simulink model "Target_Control_System"  (R2021b)
settings: Solver=FixedStepDiscrete  StartTime=0.0  StopTime=5  RelTol=1e-3
PreLoadFcn:
  | RTWConfigurationCB('preloadfcn', bdroot);
PostLoadFcn:
  | load('configuration/data_struct.mat');
  | load('configuration/fluxMaps_propMotor.mat');
  | load('configuration/parameterInit_PROP.mat');
  | load('configuration/parameterInit_PUMP.mat');
  | load('configuration/parameterInit_PITCH.mat');
  | load('configuration/parameterInit_TILT.mat');
  | %load('configuration/base_workspace_signal_definition.mat');
  | %load('resolvedatastores_to_baseworkspace_for_faster_simulation.mat');
model workspace (MAT data in the model file):
  SIMULATION_OPTIONS : Simulink.Parameter (value not decoded)
  TARGET_CODE_GEN : Simulink.Parameter (value not decoded)
  TCS_SAMPLE_FREQ_HZ : Simulink.Parameter (value not decoded)
symbols that are objects in the model workspace (value not decoded): TARGET_CODE_GEN, TCS_SAMPLE_FREQ_HZ
undefined symbols (not defined in the file): A_DQ_REF_LPF_INIT__PITCH, A_DQ_REF_LPF_INIT__PROP, A_DQ_REF_LPF_INIT__PUMP, A_DQ_REF_LPF_INIT__TILT, A_OBSERVER_CONFIDENCE_INIT__PITCH, A_OBSERVER_CONFIDENCE_INIT__PROP, A_OBSERVER_CONFIDENCE_INIT__PUMP, A_OBSERVER_CONFIDENCE_INIT__TILT, ACTUATOR_MAX_ANGLE_TRIP__PITCH, ACTUATOR_MIN_ANGLE_TRIP__PITCH, ACTUATOR_POS_SENSOR_INV_DIRECTION__PITCH, ACTUATOR_POS_SENSOR_INV_DIRECTION__TILT, ACTUATOR_POS_SENSOR_OFFSET__PITCH, ACTUATOR_POS_SENSOR_OFFSET__TILT, ADC_scaler1_baseaddr_TILT, ADC_SCALER_FLOAT_TO_FIXPOINT_EXPANSION, ANGLE_ELEC_FROM_SENSOR_OFFSET_INIT__PITCH, ANGLE_ELEC_FROM_SENSOR_OFFSET_INIT__PROP, ANGLE_ELEC_FROM_SENSOR_OFFSET_INIT__PUMP, ANGLE_ELEC_FROM_SENSOR_OFFSET_INIT__TILT, AUTO_CLEAR_FAULTS_ENABLED__PITCH, AUTO_CLEAR_FAULTS_ENABLED__PROP, AUTO_CLEAR_FAULTS_ENABLED__PUMP, AUTO_CLEAR_FAULTS_ENABLED__TILT, AUTO_CLEAR_FAULTS_WAIT_TICKS__PITCH, AUTO_CLEAR_FAULTS_WAIT_TICKS__PROP, AUTO_CLEAR_FAULTS_WAIT_TICKS__PUMP, AUTO_CLEAR_FAULTS_WAIT_TICKS__TILT, AUTO_I_ZERO_IDLE_TICKS__PITCH, AUTO_I_ZERO_IDLE_TICKS__PROP, AUTO_I_ZERO_IDLE_TICKS__PUMP, AUTO_I_ZERO_IDLE_TICKS__TILT, AUTO_I_ZERO_OFFSET_IDC_THRESHOLD__PITCH, AUTO_I_ZERO_OFFSET_IDC_THRESHOLD__PROP, AUTO_I_ZERO_OFFSET_IDC_THRESHOLD__PUMP, AUTO_I_ZERO_OFFSET_IDC_THRESHOLD__TILT, AUTO_I_ZERO_OFFSET_IPH_THRESHOLD__PITCH, AUTO_I_ZERO_OFFSET_IPH_THRESHOLD__PROP, AUTO_I_ZERO_OFFSET_IPH_THRESHOLD__PUMP, AUTO_I_ZERO_OFFSET_IPH_THRESHOLD__TILT, AUTO_SENSORLESS_SWITCHOVER_DISABLE_OMEGA, AUTO_SENSORLESS_SWITCHOVER_ENABLE_OMEGA, AUTO_SENSORLESS_SWITCHOVER_MIN_CONFIDENCE, AUXILIARY_PROTECTION_UNIT_BASEADDR__TILT, blanking_max_error_omega_INIT_PITCH, blanking_max_error_omega_INIT_TILT, blanking_max_error_position_INIT_PITCH, blanking_max_error_position_INIT_TILT, BRUTE_START_I_Q_REF_RAMP_SPEED__PITCH, BRUTE_START_I_Q_REF_RAMP_SPEED__PROP, BRUTE_START_I_Q_REF_RAMP_SPEED__PUMP, BRUTE_START_I_Q_REF_RAMP_SPEED__TILT, CONTROL_LOOP_DT_INIT__PITCH, CONTROL_LOOP_DT_INIT__PROP, CONTROL_LOOP_DT_INIT__PUMP, CONTROL_LOOP_DT_INIT__TILT, CORRECTION_FILTER_SCALE__PITCH, CORRECTION_FILTER_SCALE__PROP, CORRECTION_FILTER_SCALE__PUMP, CORRECTION_FILTER_SCALE__TILT ... (+458)
libraries: simulink x178, Reusables_Lib x24
(part 19 of 47)

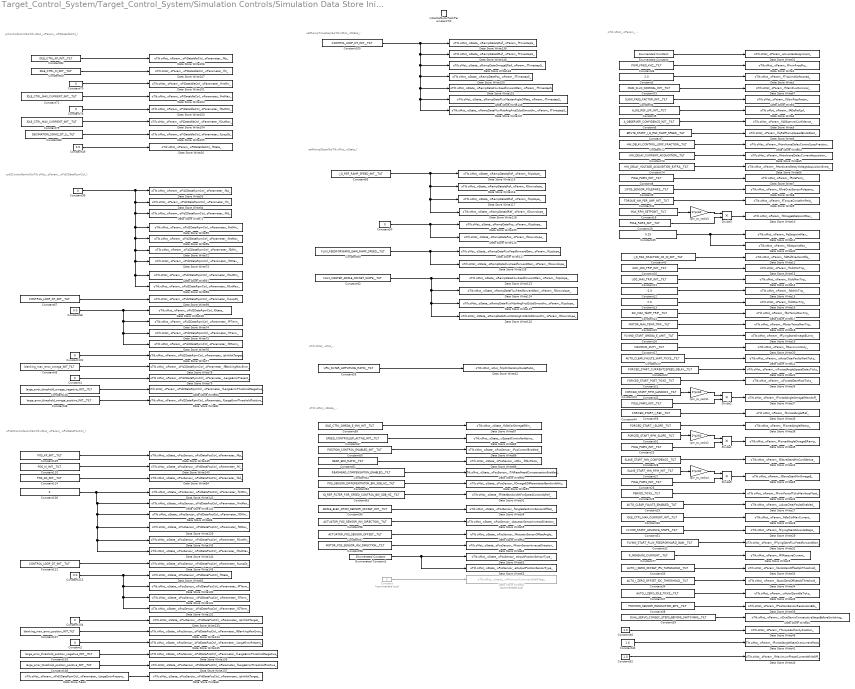
== system Target_Control_System/Target_Control_System/Simulation Controls/Simulation Data Store Initialization/initializeDataForTilt()/initializeMotorTaskParametersTilt ==
  note: oTilt.oMot_.oState_...
  note: oTilt.oMot_.oParam_...
  note: oTilt.oMot_.oOut_...
  note: setRampSlope(&oTilt.oMot_.oState_)
  note: setRampTimestep(&oTilt.oMot_.oState_)
  note: oPid2ControllerInit(&oTilt.oMot_.oParam_.oPidDataPosCtrl_)
  note: pid2ControllerInit(&oTilt.oMot_.oParam_.oPid2DataRpmCtrl_)
  note: piControllerInit(&oTilt.oMot_.oParam_.oPiDataIdleCtrl_)
  initializeMotorTaskParametersTilt : TriggerPort  TriggerType=function-call  VariantControl=Variant
  Constant : Constant  Commented=on  Value=0  OutDataTypeStr=uint32  SampleTime=-1
  Constant{1..2,101,104} (4 alike) : Constant  Value=0  OutDataTypeStr=int32  SampleTime=-1
  Constant10 : Constant  Value=UDC_MIN_TRIP_INIT__TILT  OutDataTypeStr=single  SampleTime=-1
  Constant100 : Constant  Value=large_error_threshold_omega_negative_INIT__ITLT  OutDataTypeStr=single  SampleTime=-1
  Constant103 : Constant  Value=large_error_threshold_position_negative_INIT__ITLT  OutDataTypeStr=single  SampleTime=-1
  Constant105 : Constant  Value=CONTROL_LOOP_DT_INIT__TILT  OutDataTypeStr=single  SampleTime=-1
  Constant{50,70,78,99,106} (5 alike) : Constant  Value=0  OutDataTypeStr=single  SampleTime=-1
  Constant107 : Constant  Value=blanking_max_error_position_INIT_TILT  OutDataTypeStr=single  SampleTime=-1
  Constant108 : Constant  Value=large_error_threshold_position_positive_INIT__TILT  OutDataTypeStr=single  SampleTime=-1
  Constant109 : Constant  Value=POS_KP_INIT__TILT  OutDataTypeStr=single  SampleTime=-1
  Constant11 : Constant  Value=UDC_MAX_TRIP_INIT__TILT  VectorParams1D=off  OutDataTypeStr=single  SampleTime=-1
  Constant110 : Constant  Value=POS_KI_INIT__TILT  OutDataTypeStr=single  SampleTime=-1
  Constant112 : Constant  Value=CONTROL_LOOP_DT_INIT__TILT  OutDataTypeStr=single  SampleTime=-1
  Constant113 : Constant  Value=0.0  OutDataTypeStr=single  SampleTime=-1
  Constant114 : Constant  Value=POS_KD_INIT__TILT  OutDataTypeStr=single  SampleTime=-1
  Constant12 : Constant  Value=-2.0  OutDataTypeStr=single  SampleTime=-1
  Constant13 : Constant  Value=2.0  OutDataTypeStr=single  SampleTime=-1
  Constant14 : Constant  Value=SIC_MAX_TEMP_TRIP__TILT  OutDataTypeStr=single  SampleTime=-1
  Constant15 : Constant  Value=MOTOR_MAX_TEMP_TRIP__TILT  OutDataTypeStr=single  SampleTime=-1
  Constant16 : Constant  Value=FLYING_START_OMEGA_E_LIMIT__TILT  OutDataTypeStr=single  SampleTime=-1
  Constant17 : Constant  Value=MAXIMUM_DUTY__TILT  VectorParams1D=off  OutDataTypeStr=single  SampleTime=-1
  Constant18 : Constant  Value=MAX_RPM_SETPOINT__TILT  OutDataTypeStr=single  SampleTime=-1
  Constant{8,19,23..24,26} (5 alike) : Constant  Value=POLE_PAIRS_INIT__TILT  OutDataTypeStr=single  SampleTime=-1
  Constant20 : Constant  Value=AUTO_CLEAR_FAULTS_WAIT_TICKS__TILT  OutDataTypeStr=uint32  SampleTime=-1
  Constant21 : Constant  Value=FORCED_START_POST_TICKS__TILT  OutDataTypeStr=uint32  SampleTime=-1
  Constant22 : Constant  Value=FORCED_START_CURRENT2SPEED_DELAY__TILT  OutDataTypeStr=uint32  SampleTime=-1
  Constant25 : Constant  Value=PERIOD_TICKS__TILT  OutDataTypeStr=single  SampleTime=-1
  Constant27 : Constant  Value=SLAVE_START_MIN_RPM_INIT__TILT  OutDataTypeStr=single  SampleTime=-1
  Constant28 : Constant  Value=SLAVE_START_MIN_CONFIDENCE__TILT  OutDataTypeStr=single  SampleTime=-1
  Constant29 : Constant  Value=AUTO_CLEAR_FAULTS_ENABLED__TILT  OutDataTypeStr=uint32  SampleTime=-1
  Constant3 : Constant  Value=2.0  OutDataTypeStr=single  SampleTime=-1
  Constant30 : Constant  Value=IDLE_CTRL_MAX_CURRENT_INIT__TILT  OutDataTypeStr=single  SampleTime=-1
  Constant31 : Constant  Value=FLYING_START_ADVANCE_STEPS__TILT  OutDataTypeStr=single  SampleTime=-1
  Constant32 : Constant  Value=FLYING_START_FLUX_FEEDFORWARD_GAIN__TILT  OutDataTypeStr=single  SampleTime=-1
  Constant33 : Constant  Value=AUTO_I_ZERO_OFFSET_IPH_THRESHOLD__TILT  OutDataTypeStr=single  SampleTime=-1
  Constant34 : Constant  Value=AUTO_I_ZERO_OFFSET_IDC_THRESHOLD__TILT  VectorParams1D=off  OutDataTypeStr=single  SampleTime=-1
  Constant35 : Constant  Value=0.25  VectorParams1D=off  OutDataTypeStr=single  SampleTime=-1
  Constant36 : Constant  Value=PWM_FREQ_KHZ__TILT  OutDataTypeStr=single  SampleTime=-1
  Constant37 : Constant  Value=AUTO_I_ZERO_IDLE_TICKS__TILT  OutDataTypeStr=uint32  SampleTime=-1
  Constant38 : Constant  Value=POSITION_SENSOR_RESOLUTION_BITS__TILT  OutDataTypeStr=single  SampleTime=-1
  Constant39 : Constant  Value=DUAL_SERVO_CONSEC_STEPS_BEFORE_SWITCHING__TILT  OutDataTypeStr=uint32  SampleTime=-1
  Constant4 : Constant  Value=SLOW_PASS_FACTOR_INIT__TILT  OutDataTypeStr=single  SampleTime=-1
  Constant40 : Constant  Value=1.6  OutDataTypeStr=single  SampleTime=-1
  Constant41 : Constant  Value=TORQUE_NM_PER_AMP_INIT__TILT  VectorParams1D=off  OutDataTypeStr=single  SampleTime=-1
  Constant42 : Constant  Value=FORCED_START_RPM_HANDOFF__TILT  OutDataTypeStr=single  SampleTime=-1
  Constant43 : Constant  Value=I_D_REF_FRACTION_OF_IQ_INIT__TILT  OutDataTypeStr=single  SampleTime=-1
  Constant44 : Constant  Value=FORCED_START_I_SLOPE__TILT  OutDataTypeStr=single  SampleTime=-1
  Constant45 : Constant  Value=blanking_max_error_omega_INIT_TILT  OutDataTypeStr=single  SampleTime=-1
  Constant46 : Constant  Value=1.0  OutDataTypeStr=single  SampleTime=-1
  Constant47 : Constant  Value=SPEED_CONTROLLER_ACTIVE_INIT__TILT  OutDataTypeStr=uint32  SampleTime=-1
  Constant48 : Constant  Value=large_error_threshold_omega_positive_INIT__TILT  OutDataTypeStr=single  SampleTime=-1
  Constant49 : Constant  Value=0.0  OutDataTypeStr=single  SampleTime=-1
  Constant5 : Constant  Value=A_DQ_REF_LPF_INIT__TILT  OutDataTypeStr=single  SampleTime=-1
  Constant51 : Constant  Value=FORCED_START_RPM_SLOPE__TILT  OutDataTypeStr=single  SampleTime=-1
  Constant52 : Constant  Value=1.0  OutDataTypeStr=single  SampleTime=-1
  Constant55 : Constant  Value=UPH_FILTER_AMPLITUDE_RATIO__TILT  VectorParams1D=off  OutDataTypeStr=single  SampleTime=-1
  Constant56 : Constant  Value=FORCED_START_I_REF__TILT  VectorParams1D=off  OutDataTypeStr=single  SampleTime=-1
  Constant58 : Constant  Value=IDLE_CTRL_OMEGA_E_MIN_INIT__TILT  OutDataTypeStr=single  SampleTime=-1
  Constant6 : Constant  Value=A_OBSERVER_CONFIDENCE_INIT__TILT  OutDataTypeStr=single  SampleTime=-1
  Constant60 : Constant  Value=POSITION_CONTROL_ENABLED_INIT__TILT  OutDataTypeStr=int32  SampleTime=-1
  Constant61 : Constant  Value=GEAR_BOX_RATIO__TILT  OutDataTypeStr=single  SampleTime=-1
  Constant62 : Constant  Value=READHEAD_COMPENSATION_ENABLED__TILT  OutDataTypeStr=int32  SampleTime=-1
  Constant63 : Constant  Value=IQ_REF_FILTER_FOR_SPEED_CONTROL_BW_3DB_HZ__TILT  OutDataTypeStr=single  SampleTime=-1
  Constant67 : Constant  Value=CONTROL_LOOP_DT_INIT__TILT  OutDataTypeStr=single  SampleTime=-1
  Constant68 : Constant  Value=0.0  OutDataTypeStr=single  SampleTime=-1
  Constant69 : Constant  Value=IDLE_CTRL_KI_INIT__TILT  OutDataTypeStr=single  SampleTime=-1
  Constant7 : Constant  Value=BRUTE_START_I_Q_REF_RAMP_SPEED__TILT  OutDataTypeStr=single  SampleTime=-1
  Constant71 : Constant  Value=IDLE_CTRL_MAX_CURRENT_INIT__TILT  OutDataTypeStr=single  SampleTime=-1
  Constant72 : Constant  Value=HW_DELAY_CONTROL_LOOP_FRACTION__TILT  OutDataTypeStr=single  SampleTime=-1
  Constant73 : Constant  Value=HW_DELAY_CURRENT_ACQUISITION__TILT  OutDataTypeStr=single  SampleTime=-1
  Constant74 : Constant  Value=HW_DELAY_VOLTAGE_ACQUISITION_EXTRA__TILT  OutDataTypeStr=single  SampleTime=-1
  Constant75 : Constant  Value=MAIN_FLUX_NOMINAL_INIT__TILT  OutDataTypeStr=single  SampleTime=-1
  Constant77 : Constant  Value=R_MEASURE_CURRENT__TILT  OutDataTypeStr=single  SampleTime=-1
  Constant79 : Constant  Value=IDLE_CTRL_MAX_CURRENT_INIT__TILT  VectorParams1D=off  OutDataTypeStr=single  SampleTime=-1
  Constant80 : Constant  Value=DECIMATION_200HZ_DT_S__TILT  OutDataTypeStr=single  SampleTime=-1
  Constant81 : Constant  Value=IDLE_CTRL_KP_INIT__TILT  OutDataTypeStr=single  SampleTime=-1
  Constant83 : Constant  Value=I_Q_REF_RAMP_SPEED_INIT__TILT  OutDataTypeStr=single  SampleTime=-1
  Constant89 : Constant  Value=FLUX_FEEDFORWARD_GAIN_RAMP_SPEED__TILT  OutDataTypeStr=single  SampleTime=-1
  Constant9 : Constant  Value=1/POS_SENSOR_POLEPAIRS__TILT  OutDataTypeStr=single  SampleTime=-1
  Constant92 : Constant  Value=FLUX_MASTER_ANGLE_OFFSET_SLOPE__TILT  OutDataTypeStr=single  SampleTime=-1
  Constant94 : Constant  Value=POS_SENSOR_DIFFERENTIATOR_BW_3DB_HZ__TILT  OutDataTypeStr=single  SampleTime=-1
  Constant95 : Constant  Value=ANGLE_ELEC_FROM_SENSOR_OFFSET_INIT__TILT  OutDataTypeStr=single  SampleTime=-1
  Constant96 : Constant  Value=ACTUATOR_POS_SENSOR_INV_DIRECTION__TILT  OutDataTypeStr=int32  SampleTime=-1
  Constant97 : Constant  Value=ACTUATOR_POS_SENSOR_OFFSET__TILT  OutDataTypeStr=single  SampleTime=-1
  Constant98 : Constant  Value=MOTOR_POS_SENSOR_INV_DIRECTION__TILT  OutDataTypeStr=int32  SampleTime=-1
  Data Store Read : DataStoreRead  DataStoreName=oTilt  DataStoreElements=oTilt.oMot_.oParam_.oPid2DataRpmCtrl_.oParameter_.iLargeErrorPresent_  IndexOptions=Index vector (dialog)  Indices=1  OutputSizes=1
  Data Store Write1 : DataStoreWrite  DataStoreName=oTilt  DataStoreElements=oTilt.oMot_.oParam_.fPwmFreqKhz_  IndexOptions=Index vector (dialog)  Indices=1  OutputSizes=1
  Data Store Write10 : DataStoreWrite  DataStoreName=oTilt  DataStoreElements=oTilt.oMot_.oParam_.fOmegaESetpointMax_  IndexOptions=Index vector (dialog)  Indices=1  OutputSizes=1
  Data Store Write100 : DataStoreWrite  DataStoreName=oTilt  DataStoreElements=oTilt.oMot_.oParam_.oPid2DataRpmCtrl_.fState_  IndexOptions=Index vector (dialog)  Indices=1  OutputSizes=1
  Data Store Write101 : DataStoreWrite  DataStoreName=oTilt  DataStoreElements=oTilt.oMot_.oParam_.oPiDataIdleCtrl_.oParameter_.fIntMin_  IndexOptions=Index vector (dialog)  Indices=1  OutputSizes=1
  Data Store Write102 : DataStoreWrite  DataStoreName=oTilt  DataStoreElements=oTilt.oMot_.oParam_.oPiDataIdleCtrl_.oParameter_.fIntMax_  IndexOptions=Index vector (dialog)  Indices=1  OutputSizes=1
  Data Store Write103 : DataStoreWrite  DataStoreName=oTilt  DataStoreElements=oTilt.oMot_.oParam_.oPiDataIdleCtrl_.oParameter_.fOutMin_  IndexOptions=Index vector (dialog)  Indices=1  OutputSizes=1
  Data Store Write104 : DataStoreWrite  DataStoreName=oTilt  DataStoreElements=oTilt.oMot_.oParam_.oPiDataIdleCtrl_.oParameter_.fOutMax_  IndexOptions=Index vector (dialog)  Indices=1  OutputSizes=1
  Data Store Write105 : DataStoreWrite  DataStoreName=oTilt  DataStoreElements=oTilt.oMot_.oParam_.oPiDataIdleCtrl_.oParameter_.fLoopDt_  IndexOptions=Index vector (dialog)  Indices=1  OutputSizes=1
  Data Store Write106 : DataStoreWrite  DataStoreName=oTilt  DataStoreElements=oTilt.oMot_.oParam_.oPiDataIdleCtrl_.oParameter_.fKp_  IndexOptions=Index vector (dialog)  Indices=1  OutputSizes=1
  Data Store Write107 : DataStoreWrite  DataStoreName=oTilt  DataStoreElements=oTilt.oMot_.oParam_.oPiDataIdleCtrl_.oParameter_.fKi_  IndexOptions=Index vector (dialog)  Indices=1  OutputSizes=1
  Data Store Write11 : DataStoreWrite  DataStoreName=oTilt  DataStoreElements=oTilt.oMot_.oParam_.fIqSetpointMax_  IndexOptions=Index vector (dialog)  Indices=1  OutputSizes=1
  Data Store Write115 : DataStoreWrite  DataStoreName=oTilt  DataStoreElements=oTilt.oMot_.oState_.oRampDataIqRef_.oParam_.fUpslope_  IndexOptions=Index vector (dialog)  Indices=1  OutputSizes=1
  Data Store Write116 : DataStoreWrite  DataStoreName=oTilt  DataStoreElements=oTilt.oMot_.oState_.oRampDataIqRef_.oParam_.fDownslope_  IndexOptions=Index vector (dialog)  Indices=1  OutputSizes=1
  Data Store Write117 : DataStoreWrite  DataStoreName=oTilt  DataStoreElements=oTilt.oMot_.oState_.oRampDataIdRef_.oParam_.fUpslope_  IndexOptions=Index vector (dialog)  Indices=1  OutputSizes=1
  Data Store Write118 : DataStoreWrite  DataStoreName=oTilt  DataStoreElements=oTilt.oMot_.oState_.oRampDataIdRef_.oParam_.fDownslope_  IndexOptions=Index vector (dialog)  Indices=1  OutputSizes=1
  Data Store Write119 : DataStoreWrite  DataStoreName=oTilt  DataStoreElements=oTilt.oMot_.oState_.oRampDataFluxMstrAngFrcd2clsdSmoothn_.oParam_.fUpslope_  IndexOptions=Index vector (dialog)  Indices=1  OutputSizes=1
  Data Store Write12 : DataStoreWrite  DataStoreName=oTilt  DataStoreElements=oTilt.oMot_.oParam_.fIdRefFractionOfIq_  IndexOptions=Index vector (dialog)  Indices=1  OutputSizes=1
  Data Store Write120 : DataStoreWrite  DataStoreName=oTilt  DataStoreElements=oTilt.oMot_.oState_.oRampDataFluxMstrAngFrcd2clsdSmoothn_.oParam_.fDownslope_  IndexOptions=Index vector (dialog)  Indices=1  OutputSizes=1
  Data Store Write123 : DataStoreWrite  DataStoreName=oTilt  DataStoreElements=oTilt.oMot_.oState_.oRampDataFluxFeedforwardGain_.oParam_.fUpslope_  IndexOptions=Index vector (dialog)  Indices=1  OutputSizes=1
  Data Store Write124 : DataStoreWrite  DataStoreName=oTilt  DataStoreElements=oTilt.oMot_.oState_.oRampDataFluxFeedforwardGain_.oParam_.fDownslope_  IndexOptions=Index vector (dialog)  Indices=1  OutputSizes=1
  Data Store Write125 : DataStoreWrite  DataStoreName=oTilt  DataStoreElements=oTilt.oMot_.oState_.oRampDataPos_.oParam_.fUpslope_  IndexOptions=Index vector (dialog)  Indices=1  OutputSizes=1
  Data Store Write126 : DataStoreWrite  DataStoreName=oTilt  DataStoreElements=oTilt.oMot_.oState_.oRampDataPos_.oParam_.fDownslope_  IndexOptions=Index vector (dialog)  Indices=1  OutputSizes=1
  Data Store Write127 : DataStoreWrite  DataStoreName=oTilt  DataStoreElements=oTilt.oMot_.oState_.oRampDataFluxFeedforwardGain_.oParam_.fUpslope_  IndexOptions=Index vector (dialog)  Indices=1  OutputSizes=1
  Data Store Write128 : DataStoreWrite  DataStoreName=oTilt  DataStoreElements=oTilt.oMot_.oState_.oRampDataFluxFeedforwardGain_.oParam_.fDownslope_  IndexOptions=Index vector (dialog)  Indices=1  OutputSizes=1
  Data Store Write129 : DataStoreWrite  DataStoreName=oTilt  DataStoreElements=oTilt.oMot_.oState_.oPosSensor_.oPidDataPosCtrl_.oParameter_.fDMax_  IndexOptions=Index vector (dialog)  Indices=1  OutputSizes=1
  Data Store Write13 : DataStoreWrite  DataStoreName=oTilt  DataStoreElements=oTilt.oMot_.oParam_.fUdcMinTrip_  IndexOptions=Index vector (dialog)  Indices=1  OutputSizes=1
  Data Store Write130 : DataStoreWrite  DataStoreName=oTilt  DataStoreElements=oTilt.oMot_.oState_.oPosSensor_.oPidDataPosCtrl_.oParameter_.fPTerm_  IndexOptions=Index vector (dialog)  Indices=1  OutputSizes=1
  Data Store Write131 : DataStoreWrite  DataStoreName=oTilt  DataStoreElements=oTilt.oMot_.oState_.oPosSensor_.oPidDataPosCtrl_.oParameter_.fITerm_  IndexOptions=Index vector (dialog)  Indices=1  OutputSizes=1
  Data Store Write132 : DataStoreWrite  DataStoreName=oTilt  DataStoreElements=oTilt.oMot_.oState_.oPosSensor_.oPidDataPosCtrl_.oParameter_.fDTerm_  IndexOptions=Index vector (dialog)  Indices=1  OutputSizes=1
  Data Store Write133 : DataStoreWrite  DataStoreName=oTilt  DataStoreElements=oTilt.oMot_.oState_.oPosSensor_.oPidDataPosCtrl_.oParameter_.ipInhibitTarget_  IndexOptions=Index vector (dialog)  Indices=1  OutputSizes=1
  Data Store Write134 : DataStoreWrite  DataStoreName=oTilt  DataStoreElements=oTilt.oMot_.oState_.oPosSensor_.oPidDataPosCtrl_.oParameter_.fBlankingMaxError_  IndexOptions=Index vector (dialog)  Indices=1  OutputSizes=1
  Data Store Write135 : DataStoreWrite  DataStoreName=oTilt  DataStoreElements=oTilt.oMot_.oState_.oPosSensor_.oPidDataPosCtrl_.oParameter_.iLargeErrorPresent_  IndexOptions=Index vector (dialog)  Indices=1  OutputSizes=1
  Data Store Write136 : DataStoreWrite  DataStoreName=oTilt  DataStoreElements=oTilt.oMot_.oState_.oPosSensor_.oPidDataPosCtrl_.oParameter_.fLargeErrorThresholdNegative_  IndexOptions=Index vector (dialog)  Indices=1  OutputSizes=1
  Data Store Write137 : DataStoreWrite  DataStoreName=oTilt  DataStoreElements=oTilt.oMot_.oState_.oPosSensor_.oPidDataPosCtrl_.oParameter_.fLargeErrorThresholdPositive_  IndexOptions=Index vector (dialog)  Indices=1  OutputSizes=1
  Data Store Write138 : DataStoreWrite  DataStoreName=oTilt  DataStoreElements=oTilt.oMot_.oState_.oRampDataIqRef_.oParam_.fTimestepS_  IndexOptions=Index vector (dialog)  Indices=1  OutputSizes=1
  Data Store Write139 : DataStoreWrite  DataStoreName=oTilt  DataStoreElements=oTilt.oMot_.oState_.oPosSensor_.oPidDataPosCtrl_.oParameter_.fKp_  IndexOptions=Index vector (dialog)  Indices=1  OutputSizes=1
  Data Store Write14 : DataStoreWrite  DataStoreName=oTilt  DataStoreElements=oTilt.oMot_.oParam_.fUdcMaxTrip_  IndexOptions=Index vector (dialog)  Indices=1  OutputSizes=1
  Data Store Write140 : DataStoreWrite  DataStoreName=oTilt  DataStoreElements=oTilt.oMot_.oState_.oPosSensor_.oPidDataPosCtrl_.oParameter_.fKi_  IndexOptions=Index vector (dialog)  Indices=1  OutputSizes=1
  Data Store Write141 : DataStoreWrite  DataStoreName=oTilt  DataStoreElements=oTilt.oMot_.oState_.oPosSensor_.oPidDataPosCtrl_.oParameter_.fIntMin_  IndexOptions=Index vector (dialog)  Indices=1  OutputSizes=1
  Data Store Write142 : DataStoreWrite  DataStoreName=oTilt  DataStoreElements=oTilt.oMot_.oState_.oPosSensor_.oPidDataPosCtrl_.oParameter_.fIntMax_  IndexOptions=Index vector (dialog)  Indices=1  OutputSizes=1
  Data Store Write143 : DataStoreWrite  DataStoreName=oTilt  DataStoreElements=oTilt.oMot_.oState_.oPosSensor_.oPidDataPosCtrl_.oParameter_.fOutMin_  IndexOptions=Index vector (dialog)  Indices=1  OutputSizes=1
  Data Store Write144 : DataStoreWrite  DataStoreName=oTilt  DataStoreElements=oTilt.oMot_.oState_.oPosSensor_.oPidDataPosCtrl_.oParameter_.fOutMax_  IndexOptions=Index vector (dialog)  Indices=1  OutputSizes=1
  Data Store Write145 : DataStoreWrite  DataStoreName=oTilt  DataStoreElements=oTilt.oMot_.oState_.oPosSensor_.oPidDataPosCtrl_.oParameter_.fLoopDt_  IndexOptions=Index vector (dialog)  Indices=1  OutputSizes=1
  Data Store Write146 : DataStoreWrite  DataStoreName=oTilt  DataStoreElements=oTilt.oMot_.oState_.oRampDataIdRef_.oParam_.fTimestepS_  IndexOptions=Index vector (dialog)  Indices=1  OutputSizes=1
  Data Store Write147 : DataStoreWrite  DataStoreName=oTilt  DataStoreElements=oTilt.oMot_.oState_.oRampDataFluxMstrAngFrcd2clsdSmoothn_.oParam_.fTimestepS_  IndexOptions=Index vector (dialog)  Indices=1  OutputSizes=1
  Data Store Write148 : DataStoreWrite  DataStoreName=oTilt  DataStoreElements=oTilt.oMot_.oState_.oRampDataOmegaERef_.oParam_.fTimestepS_  IndexOptions=Index vector (dialog)  Indices=1  OutputSizes=1
  Data Store Write149 : DataStoreWrite  DataStoreName=oTilt  DataStoreElements=oTilt.oMot_.oState_.oRampDataFluxMasterAngleOffset_.oParam_.fTimestepS_  IndexOptions=Index vector (dialog)  Indices=1  OutputSizes=1
  Data Store Write15 : DataStoreWrite  DataStoreName=oTilt  DataStoreElements=oTilt.oMot_.oParam_.fIdcMinTrip_  IndexOptions=Index vector (dialog)  Indices=1  OutputSizes=1
  Data Store Write150 : DataStoreWrite  DataStoreName=oTilt  DataStoreElements=oTilt.oMot_.oState_.oRampDataPos_.oParam_.fTimestepS_  IndexOptions=Index vector (dialog)  Indices=1  OutputSizes=1
  Data Store Write151 : DataStoreWrite  DataStoreName=oTilt  DataStoreElements=oTilt.oMot_.oState_.oRampDataFluxFeedforwardGain_.oParam_.fTimestepS_  IndexOptions=Index vector (dialog)  Indices=1  OutputSizes=1
  Data Store Write16 : DataStoreWrite  DataStoreName=oTilt  DataStoreElements=oTilt.oMot_.oParam_.fIdcMaxTrip_  IndexOptions=Index vector (dialog)  Indices=1  OutputSizes=1
  Data Store Write17 : DataStoreWrite  DataStoreName=oTilt  DataStoreElements=oTilt.oMot_.oParam_.fSicTempMaxTrip_  IndexOptions=Index vector (dialog)  Indices=1  OutputSizes=1
  Data Store Write18 : DataStoreWrite  DataStoreName=oTilt  DataStoreElements=oTilt.oMot_.oParam_.fMotorTempMaxTrip_  IndexOptions=Index vector (dialog)  Indices=1  OutputSizes=1
  Data Store Write19 : DataStoreWrite  DataStoreName=oTilt  DataStoreElements=oTilt.oMot_.oParam_.fFlyingStartOmegaELimit_  IndexOptions=Index vector (dialog)  Indices=1  OutputSizes=1
  Data Store Write2 : DataStoreWrite  DataStoreName=oTilt  DataStoreElements=oTilt.oMot_.oParam_.fTripLimitSoftwareA_  IndexOptions=Index vector (dialog)  Indices=1  OutputSizes=1
  Data Store Write20 : DataStoreWrite  DataStoreName=oTilt  DataStoreElements=oTilt.oMot_.oParam_.fMaximumDuty_  IndexOptions=Index vector (dialog)  Indices=1  OutputSizes=1
  Data Store Write21 : DataStoreWrite  DataStoreName=oTilt  DataStoreElements=oTilt.oMot_.oParam_.uiAutoClearFaultsWaitTicks_  IndexOptions=Index vector (dialog)  Indices=1  OutputSizes=1
  Data Store Write22 : DataStoreWrite  DataStoreName=oTilt  DataStoreElements=oTilt.oMot_.oParam_.uiForcedAngleSpeedDelayTicks_  IndexOptions=Index vector (dialog)  Indices=1  OutputSizes=1
  Data Store Write23 : DataStoreWrite  DataStoreName=oTilt  DataStoreElements=oTilt.oMot_.oParam_.fSlaveStartMinConfidence_  IndexOptions=Index vector (dialog)  Indices=1  OutputSizes=1
  Data Store Write24 : DataStoreWrite  DataStoreName=oTilt  DataStoreElements=oTilt.oMot_.oParam_.fPwmPeriodTicksMainloopFloat_  IndexOptions=Index vector (dialog)  Indices=1  OutputSizes=1
  Data Store Write25 : DataStoreWrite  DataStoreName=oTilt  DataStoreElements=oTilt.oMot_.oParam_.fRMeasureCurrent_  IndexOptions=Index vector (dialog)  Indices=1  OutputSizes=1
  Data Store Write26 : DataStoreWrite  DataStoreName=oTilt  DataStoreElements=oTilt.oMot_.oParam_.oPiDataIdleCtrl_.fState_  IndexOptions=Index vector (dialog)  Indices=1  OutputSizes=1
  Data Store Write27 : DataStoreWrite  DataStoreName=oTilt  DataStoreElements=oTilt.oMot_.oParam_.uiAutoClearFaultsEnabled_  IndexOptions=Index vector (dialog)  Indices=1  OutputSizes=1
  Data Store Write28 : DataStoreWrite  DataStoreName=oTilt  DataStoreElements=oTilt.oMot_.oParam_.fIdleCtrlMaxCurrent_  IndexOptions=Index vector (dialog)  Indices=1  OutputSizes=1
  Data Store Write29 : DataStoreWrite  DataStoreName=oTilt  DataStoreElements=oTilt.oMot_.oParam_.fFlyingStartAdvanceSteps_  IndexOptions=Index vector (dialog)  Indices=1  OutputSizes=1
  Data Store Write3 : DataStoreWrite  DataStoreName=oTilt  DataStoreElements=oTilt.oMot_.oParam_.fSlowPassFactor_  IndexOptions=Index vector (dialog)  Indices=1  OutputSizes=1
  Data Store Write30 : DataStoreWrite  DataStoreName=oTilt  DataStoreElements=oTilt.oMot_.oParam_.fISetpointMax_  IndexOptions=Index vector (dialog)  Indices=1  OutputSizes=1
  Data Store Write31 : DataStoreWrite  DataStoreName=oTilt  DataStoreElements=oTilt.oMot_.oParam_.eInverterAssignment_  IndexOptions=Index vector (dialog)  Indices=1  OutputSizes=1
  Data Store Write32 : DataStoreWrite  DataStoreName=oTilt  DataStoreElements=oTilt.oMot_.oParam_.fFlyingStartFluxFeedforwardGain_  IndexOptions=Index vector (dialog)  Indices=1  OutputSizes=1
  Data Store Write33 : DataStoreWrite  DataStoreName=oTilt  DataStoreElements=oTilt.oMot_.oParam_.fAutoIZeroOffsetIphThreshold_  IndexOptions=Index vector (dialog)  Indices=1  OutputSizes=1
  Data Store Write34 : DataStoreWrite  DataStoreName=oTilt  DataStoreElements=oTilt.oMot_.oParam_.fAutoIZeroOffsetIdcThreshold_  IndexOptions=Index vector (dialog)  Indices=1  OutputSizes=1
  Data Store Write35 : DataStoreWrite  DataStoreName=oTilt  DataStoreElements=oTilt.oMot_.oParam_.uiAutoIZeroIdleTicks_  IndexOptions=Index vector (dialog)  Indices=1  OutputSizes=1
  Data Store Write36 : DataStoreWrite  DataStoreName=oTilt  DataStoreElements=oTilt.oMot_.oParam_.uiForcedStartPostTicks_  IndexOptions=Index vector (dialog)  Indices=1  OutputSizes=1
  Data Store Write37 : DataStoreWrite  DataStoreName=oTilt  DataStoreElements=oTilt.oMot_.oParam_.fForcedAngleOmegaEHandoff_  IndexOptions=Index vector (dialog)  Indices=1  OutputSizes=1
  Data Store Write38 : DataStoreWrite  DataStoreName=oTilt  DataStoreElements=oTilt.oMot_.oParam_.fForcedAngleIRamp_  IndexOptions=Index vector (dialog)  Indices=1  OutputSizes=1
  Data Store Write39 : DataStoreWrite  DataStoreName=oTilt  DataStoreElements=oTilt.oMot_.oParam_.fPositionSensorResolutionBits_  IndexOptions=Index vector (dialog)  Indices=1  OutputSizes=1
  Data Store Write4 : DataStoreWrite  DataStoreName=oTilt  DataStoreElements=oTilt.oMot_.oParam_.fADqRefLpf_  IndexOptions=Index vector (dialog)  Indices=1  OutputSizes=1
  Data Store Write40 : DataStoreWrite  DataStoreName=oTilt  DataStoreElements=oTilt.oMot_.oParam_.uiDualServoConsecutiveStepsBeforeSwitching_  IndexOptions=Index vector (dialog)  Indices=1  OutputSizes=1
  Data Store Write41 : DataStoreWrite  DataStoreName=oTilt  DataStoreElements=oTilt.oMot_.oParam_.fForcedAngleStartOvercurrentRatio_  IndexOptions=Index vector (dialog)  Indices=1  OutputSizes=1
  Data Store Write42 : DataStoreWrite  DataStoreName=oTilt  DataStoreElements=oTilt.oMot_.oOut_.fUphFilterAmplitudeRatio_  IndexOptions=Index vector (dialog)  Indices=1  OutputSizes=1
  Data Store Write43 : DataStoreWrite  DataStoreName=oTilt  DataStoreElements=oTilt.oMot_.oParam_.fMaximumPhaseCurrentWhileOff_  IndexOptions=Index vector (dialog)  Indices=1  OutputSizes=1
  Data Store Write45 : DataStoreWrite  DataStoreName=oTilt  DataStoreElements=oTilt.oMot_.oParam_.fForcedAngleOmegaERamp_  IndexOptions=Index vector (dialog)  Indices=1  OutputSizes=1
  Data Store Write46 : DataStoreWrite  DataStoreName=oTilt  DataStoreElements=oTilt.oMot_.oParam_.fTorqueAuthorityFraction_  IndexOptions=Index vector (dialog)  Indices=1  OutputSizes=1
  Data Store Write49 : DataStoreWrite  DataStoreName=oTilt  DataStoreElements=oTilt.oMot_.oParam_.fForcedAngleIRef_  IndexOptions=Index vector (dialog)  Indices=1  OutputSizes=1
  Data Store Write5 : DataStoreWrite  DataStoreName=oTilt  DataStoreElements=oTilt.oMot_.oParam_.fAObserverConfidence_  IndexOptions=Index vector (dialog)  Indices=1  OutputSizes=1
  Data Store Write55 : DataStoreWrite  DataStoreName=oTilt  DataStoreElements=oTilt.oMot_.oState_.oPosSensor_.fOmegaEDifferentiatorBandwidthHz_  IndexOptions=Index vector (dialog)  Indices=1  OutputSizes=1
  Data Store Write58 : DataStoreWrite  DataStoreName=oTilt  DataStoreElements=oTilt.oMot_.oState_.oPosSensor_.fAngleElecFromSensorOffset_  IndexOptions=Index vector (dialog)  Indices=1  OutputSizes=1
  Data Store Write59 : DataStoreWrite  DataStoreName=oTilt  DataStoreElements=oTilt.oMot_.oState_.oPosSensor_.iActuatorSensorInverseDirection_  IndexOptions=Index vector (dialog)  Indices=1  OutputSizes=1
  Data Store Write6 : DataStoreWrite  DataStoreName=oTilt  DataStoreElements=oTilt.oMot_.oParam_.fIqRefRampSpeedBruteStart_  IndexOptions=Index vector (dialog)  Indices=1  OutputSizes=1
  Data Store Write60 : DataStoreWrite  DataStoreName=oTilt  DataStoreElements=oTilt.oMot_.oState_.oPosSensor_.fActuatorSensorOffsetAngle_  IndexOptions=Index vector (dialog)  Indices=1  OutputSizes=1
  Data Store Write61 : DataStoreWrite  DataStoreName=oTilt  DataStoreElements=oTilt.oMot_.oState_.oPosSensor_.iMotorSensorInverseDirection_  IndexOptions=Index vector (dialog)  Indices=1  OutputSizes=1
  Data Store Write62 : DataStoreWrite  DataStoreName=oTilt  DataStoreElements=oTilt.oMot_.oState_.oPosSensor_.eInputPositionSensorType_  IndexOptions=Index vector (dialog)  Indices=1  OutputSizes=1
  Data Store Write63 : DataStoreWrite  DataStoreName=oTilt  DataStoreElements=oTilt.oMot_.oState_.oPosSensor_.eOutputPositionSensorType_  IndexOptions=Index vector (dialog)  Indices=1  OutputSizes=1
  Data Store Write64 : DataStoreWrite  DataStoreName=oTilt  DataStoreElements=oTilt.oMot_.oParam_.fHardwareDelayControlLoopFraction_  IndexOptions=Index vector (dialog)  Indices=1  OutputSizes=1
  Data Store Write65 : DataStoreWrite  DataStoreName=oTilt  DataStoreElements=oTilt.oMot_.oParam_.fHardwareDelayCurrentAcquisition_  IndexOptions=Index vector (dialog)  Indices=1  OutputSizes=1
  Data Store Write66 : DataStoreWrite  DataStoreName=oTilt  DataStoreElements=oTilt.oMot_.oParam_.fHardwareDelayVoltageAcquisitionExtra_  IndexOptions=Index vector (dialog)  Indices=1  OutputSizes=1
  Data Store Write67 : DataStoreWrite  DataStoreName=oTilt  DataStoreElements=oTilt.oMot_.oParam_.fMainFluxNominal_  IndexOptions=Index vector (dialog)  Indices=1  OutputSizes=1
  Data Store Write68 : DataStoreWrite  DataStoreName=oTilt  DataStoreElements=oTilt.oMot_.oState_.oPosSensor_.oPidDataPosCtrl_.oParameter_.ipInhibitTarget_  IndexOptions=Index vector (dialog)  Indices=1  OutputSizes=1
  Data Store Write69 : DataStoreWrite  DataStoreName=oTilt  DataStoreElements=oTilt.oMot_.oParam_.fSlaveStartMinOmegaE_  IndexOptions=Index vector (dialog)  Indices=1  OutputSizes=1
  Data Store Write7 : DataStoreWrite  DataStoreName=oTilt  DataStoreElements=oTilt.oMot_.oParam_.fPolePairs_  IndexOptions=Index vector (dialog)  Indices=1  OutputSizes=1
  Data Store Write71 : DataStoreWrite  DataStoreName=oTilt  DataStoreElements=oTilt.oMot_.oParam_.oPid2DataRpmCtrl_.oParameter_.fKd_  IndexOptions=Index vector (dialog)  Indices=1  OutputSizes=1
  Data Store Write72 : DataStoreWrite  DataStoreName=oTilt  DataStoreElements=oTilt.oMot_.oParam_.oPid2DataRpmCtrl_.oParameter_.fDMin_  IndexOptions=Index vector (dialog)  Indices=1  OutputSizes=1
  Data Store Write73 : DataStoreWrite  DataStoreName=oTilt  DataStoreElements=oTilt.oMot_.oParam_.oPid2DataRpmCtrl_.oParameter_.fDMax_  IndexOptions=Index vector (dialog)  Indices=1  OutputSizes=1
  Data Store Write74 : DataStoreWrite  DataStoreName=oTilt  DataStoreElements=oTilt.oMot_.oParam_.oPid2DataRpmCtrl_.oParameter_.fPTerm_  IndexOptions=Index vector (dialog)  Indices=1  OutputSizes=1
  Data Store Write75 : DataStoreWrite  DataStoreName=oTilt  DataStoreElements=oTilt.oMot_.oParam_.oPid2DataRpmCtrl_.oParameter_.fITerm_  IndexOptions=Index vector (dialog)  Indices=1  OutputSizes=1
  Data Store Write76 : DataStoreWrite  DataStoreName=oTilt  DataStoreElements=oTilt.oMot_.oParam_.oPid2DataRpmCtrl_.oParameter_.fDTerm_  IndexOptions=Index vector (dialog)  Indices=1  OutputSizes=1
  Data Store Write77 : DataStoreWrite  DataStoreName=oTilt  DataStoreElements=oTilt.oMot_.oParam_.oPid2DataRpmCtrl_.oParameter_.ipInhibitTarget_  IndexOptions=Index vector (dialog)  Indices=1  OutputSizes=1
  Data Store Write78 : DataStoreWrite  DataStoreName=oTilt  DataStoreElements=oTilt.oMot_.oParam_.oPid2DataRpmCtrl_.oParameter_.fBlankingMaxError_  IndexOptions=Index vector (dialog)  Indices=1  OutputSizes=1
  Data Store Write79 : DataStoreWrite  DataStoreName=oTilt  DataStoreElements=oTilt.oMot_.oParam_.oPid2DataRpmCtrl_.oParameter_.iLargeErrorPresent_  IndexOptions=Index vector (dialog)  Indices=1  OutputSizes=1
  Data Store Write8 : DataStoreWrite  DataStoreName=oTilt  DataStoreElements=oTilt.oMot_.oParam_.fOneOverSensorPolepairs_  IndexOptions=Index vector (dialog)  Indices=1  OutputSizes=1
  Data Store Write80 : DataStoreWrite  DataStoreName=oTilt  DataStoreElements=oTilt.oMot_.oParam_.oPid2DataRpmCtrl_.oParameter_.fLargeErrorThresholdNegative_  IndexOptions=Index vector (dialog)  Indices=1  OutputSizes=1
  Data Store Write81 : DataStoreWrite  DataStoreName=oTilt  DataStoreElements=oTilt.oMot_.oParam_.oPid2DataRpmCtrl_.oParameter_.fLargeErrorThresholdPositive_  IndexOptions=Index vector (dialog)  Indices=1  OutputSizes=1
  Data Store Write83 : DataStoreWrite  DataStoreName=oTilt  DataStoreElements=oTilt.oMot_.oState_.oPosSensor_.oPidDataPosCtrl_.fState_  IndexOptions=Index vector (dialog)  Indices=1  OutputSizes=1
  Data Store Write84 : DataStoreWrite  DataStoreName=oTilt  DataStoreElements=oTilt.oMot_.oState_.oPosSensor_.oPidDataPosCtrl_.oParameter_.fKd_  IndexOptions=Index vector (dialog)  Indices=1  OutputSizes=1
  Data Store Write85 : DataStoreWrite  DataStoreName=oTilt  DataStoreElements=oTilt.oMot_.oState_.uiSpeedControllerActive_  IndexOptions=Index vector (dialog)  Indices=1  OutputSizes=1
  Data Store Write86 : DataStoreWrite  DataStoreName=oTilt  DataStoreElements=oTilt.oMot_.oState_.oPosSensor_.oPidDataPosCtrl_.oParameter_.fDMin_  IndexOptions=Index vector (dialog)  Indices=1  OutputSizes=1
  Data Store Write87 : DataStoreWrite  DataStoreName=oTilt  DataStoreElements=oTilt.oMot_.oState_.fIdleCtrlOmegaEMin_  IndexOptions=Index vector (dialog)  Indices=1  OutputSizes=1
  Data Store Write88 : DataStoreWrite  DataStoreName=oTilt  DataStoreElements=oTilt.oMot_.oState_.oPosSensor_.iPosControlEnabled_  IndexOptions=Index vector (dialog)  Indices=1  OutputSizes=1
  Data Store Write89 : DataStoreWrite  DataStoreName=oTilt  DataStoreElements=oTilt.oMot_.oState_.oPosSensor_.oGbx_.fGbxRatio_  IndexOptions=Index vector (dialog)  Indices=1  OutputSizes=1
  Data Store Write9 : DataStoreWrite  DataStoreName=oTilt  DataStoreElements=oTilt.oMot_.oParam_.fTorqueConstNmPerA_  IndexOptions=Index vector (dialog)  Indices=1  OutputSizes=1
  Data Store Write90 : DataStoreWrite  DataStoreName=oTilt  DataStoreElements=oTilt.oMot_.oState_.oPosSensor_.iTiltReadheadCompensationEnabled_  IndexOptions=Index vector (dialog)  Indices=1  OutputSizes=1
  Data Store Write91 : DataStoreWrite  DataStoreName=oTilt  DataStoreElements=oTilt.oMot_.oState_.fFilterBandwidthForSpeedControlIqRef_  IndexOptions=Index vector (dialog)  Indices=1  OutputSizes=1
  Data Store Write92 : DataStoreWrite  Commented=on  DataStoreName=oTilt  DataStoreElements=oTilt.oMot_.oState_.uiMinimumCommandSetFlags_  IndexOptions=Index vector (dialog)  Indices=1  OutputSizes=1
  Data Store Write93 : DataStoreWrite  DataStoreName=oTilt  DataStoreElements=oTilt.oMot_.oParam_.oPid2DataRpmCtrl_.oParameter_.fKp_  IndexOptions=Index vector (dialog)  Indices=1  OutputSizes=1
  Data Store Write94 : DataStoreWrite  DataStoreName=oTilt  DataStoreElements=oTilt.oMot_.oParam_.oPid2DataRpmCtrl_.oParameter_.fKi_  IndexOptions=Index vector (dialog)  Indices=1  OutputSizes=1
  Data Store Write95 : DataStoreWrite  DataStoreName=oTilt  DataStoreElements=oTilt.oMot_.oParam_.oPid2DataRpmCtrl_.oParameter_.fIntMin_  IndexOptions=Index vector (dialog)  Indices=1  OutputSizes=1
  Data Store Write96 : DataStoreWrite  DataStoreName=oTilt  DataStoreElements=oTilt.oMot_.oParam_.oPid2DataRpmCtrl_.oParameter_.fIntMax_  IndexOptions=Index vector (dialog)  Indices=1  OutputSizes=1
  Data Store Write97 : DataStoreWrite  DataStoreName=oTilt  DataStoreElements=oTilt.oMot_.oParam_.oPid2DataRpmCtrl_.oParameter_.fOutMin_  IndexOptions=Index vector (dialog)  Indices=1  OutputSizes=1
  Data Store Write98 : DataStoreWrite  DataStoreName=oTilt  DataStoreElements=oTilt.oMot_.oParam_.oPid2DataRpmCtrl_.oParameter_.fOutMax_  IndexOptions=Index vector (dialog)  Indices=1  OutputSizes=1
  Data Store Write99 : DataStoreWrite  DataStoreName=oTilt  DataStoreElements=oTilt.oMot_.oParam_.oPid2DataRpmCtrl_.oParameter_.fLoopDt_  IndexOptions=Index vector (dialog)  Indices=1  OutputSizes=1
  Divide{1..3,5} (4 alike) : Product  Inputs=**  OutDataTypeStr=single
  Enumerated Constant : simulink/Sources/Enumerated Constant  OutDataTypeStr=Enum: EInverterNames_t  Value=EInverterNames_t.eTilt  SampleTime=-1
  Enumerated Constant1 : simulink/Sources/Enumerated Constant  OutDataTypeStr=Enum: EPositionSensor_t  Value=EPositionSensor_t.eAksim2  SampleTime=-1
  rpm_to_rad/s{1..4} (4 alike) : Gain  Gain=2*pi/60  OutDataTypeStr=single
  wires:
  Constant52/1 -> Data Store Write43/1
  Constant47/1 -> Data Store Write85/1
  Constant60/1 -> Data Store Write88/1
  Constant/1 -> Data Store Write92/1
  Constant96/1 -> Data Store Write59/1
  Constant61/1 -> Data Store Write89/1
  Constant95/1 -> Data Store Write58/1
  Constant58/1 -> Data Store Write87/1
  Constant97/1 -> Data Store Write60/1
  Constant98/1 -> Data Store Write61/1
  Constant63/1 -> Data Store Write91/1
  Constant94/1 -> Data Store Write55/1
  Constant62/1 -> Data Store Write90/1
  Enumerated Constant1/1 -> Data Store Write62/1, Data Store Write63/1
  Constant51/1 -> rpm_to_rad/s2/1
  Constant39/1 -> Data Store Write40/1
  Constant20/1 -> Data Store Write21/1
  Constant5/1 -> Data Store Write4/1
  Constant19/1 -> Divide3/2
  Constant17/1 -> Data Store Write20/1
  Constant34/1 -> Data Store Write34/1
  Constant27/1 -> rpm_to_rad/s4/1
  rpm_to_rad/s1/1 -> Divide2/1
  Constant42/1 -> rpm_to_rad/s1/1
  Constant46/1 -> Data Store Write46/1
  Constant15/1 -> Data Store Write18/1
  Constant16/1 -> Data Store Write19/1
  Divide3/1 -> Data Store Write10/1
  Constant3/1 -> Data Store Write2/1
  Constant18/1 -> rpm_to_rad/s3/1
  Constant41/1 -> Data Store Write9/1
  Constant44/1 -> Data Store Write38/1
  Constant33/1 -> Data Store Write33/1
  Divide1/1 -> Data Store Write45/1
  Constant43/1 -> Data Store Write12/1
  Constant4/1 -> Data Store Write3/1
  Constant30/1 -> Data Store Write28/1
  Constant56/1 -> Data Store Write49/1
  Constant25/1 -> Data Store Write24/1
  Constant77/1 -> Data Store Write25/1
  Constant73/1 -> Data Store Write65/1
  Constant14/1 -> Data Store Write17/1
  Constant8/1 -> Data Store Write7/1
  Constant10/1 -> Data Store Write13/1
  Constant13/1 -> Data Store Write16/1
  Constant23/1 -> Divide1/2
  Constant26/1 -> Divide5/2
  Constant6/1 -> Data Store Write5/1
  rpm_to_rad/s3/1 -> Divide3/1
  Constant22/1 -> Data Store Write22/1
  Constant36/1 -> Data Store Write1/1
  Constant40/1 -> Data Store Write41/1
  Constant9/1 -> Data Store Write8/1
  rpm_to_rad/s2/1 -> Divide1/1
  Constant24/1 -> Divide2/2
  Constant37/1 -> Data Store Write35/1
  Constant32/1 -> Data Store Write32/1
  Divide5/1 -> Data Store Write69/1
  Divide2/1 -> Data Store Write37/1
  Constant75/1 -> Data Store Write67/1
  Constant38/1 -> Data Store Write39/1
  Constant28/1 -> Data Store Write23/1
  Constant12/1 -> Data Store Write15/1
  Constant74/1 -> Data Store Write66/1
  Constant31/1 -> Data Store Write29/1
  Constant11/1 -> Data Store Write14/1
  rpm_to_rad/s4/1 -> Divide5/1
  Constant72/1 -> Data Store Write64/1
  Enumerated Constant/1 -> Data Store Write31/1
  Constant7/1 -> Data Store Write6/1
  Constant35/1 -> Data Store Write30/1, Data Store Write11/1
  Constant21/1 -> Data Store Write36/1
  Constant29/1 -> Data Store Write27/1
  Constant55/1 -> Data Store Write42/1
  Constant89/1 -> Data Store Write127/1, Data Store Write128/1
  Constant50/1 -> Data Store Write125/1, Data Store Write126/1
  Constant92/1 -> Data Store Write123/1, Data Store Write120/1, Data Store Write119/1, Data Store Write124/1
  Constant83/1 -> Data Store Write115/1, Data Store Write118/1, Data Store Write117/1, Data Store Write116/1
  Constant105/1 -> Data Store Write147/1, Data Store Write149/1, Data Store Write151/1, Data Store Write150/1, Data Store Write148/1, Data Store Write146/1, Data Store Write138/1
  Constant2/1 -> Data Store Write135/1
  Constant113/1 -> Data Store Write83/1, Data Store Write130/1, Data Store Write132/1, Data Store Write131/1
  Constant109/1 -> Data Store Write139/1
  Constant107/1 -> Data Store Write134/1
  Constant106/1 -> Data Store Write141/1, Data Store Write142/1, Data Store Write86/1, Data Store Write129/1, Data Store Write143/1, Data Store Write144/1
  Constant103/1 -> Data Store Write136/1
  Constant112/1 -> Data Store Write145/1
  Constant108/1 -> Data Store Write137/1
  Constant110/1 -> Data Store Write140/1
  Constant104/1 -> Data Store Write133/1
  Constant114/1 -> Data Store Write84/1
  Data Store Read/1 -> Data Store Write68/1
  Constant1/1 -> Data Store Write79/1
  Constant68/1 -> Data Store Write100/1, Data Store Write74/1, Data Store Write76/1, Data Store Write75/1
  Constant101/1 -> Data Store Write77/1
  Constant45/1 -> Data Store Write78/1
  Constant67/1 -> Data Store Write99/1
  Constant99/1 -> Data Store Write93/1, Data Store Write71/1, Data Store Write98/1, Data Store Write97/1, Data Store Write73/1, Data Store Write72/1, Data Store Write96/1, Data Store Write95/1, Data Store Write94/1
  Constant100/1 -> Data Store Write80/1
  Constant48/1 -> Data Store Write81/1
  Constant80/1 -> Data Store Write105/1
  Constant49/1 -> Data Store Write26/1
  Constant71/1 -> Data Store Write102/1
  Constant69/1 -> Data Store Write107/1
  Constant78/1 -> Data Store Write103/1
  Constant79/1 -> Data Store Write104/1
  Constant81/1 -> Data Store Write106/1
  Constant70/1 -> Data Store Write101/1

== system Target_Control_System/Target_Control_System/Simulation Controls/Simulation Data Store Initialization/parameter_init_prop/initializeHardwareInvPropulsion() ==
  Constant1 : Constant  Value=DEADTIME_NS__PROP  OutDataTypeStr=single  SampleTime=-1
  Constant10 : Constant  Value=PHASE_CURRENT_SUM_MAX_IMBALANCE__PROP  VectorParams1D=off  OutDataTypeStr=single  SampleTime=-1
  Constant11 : Constant  Value=MAX_IDENTICAL_SAMPLES_PHASE_CURRENT__PROP  VectorParams1D=off  OutDataTypeStr=int32  SampleTime=-1
  Constant2 : Constant  Value=IIR_UPHASE_F_INIT__PROP  OutDataTypeStr=single  SampleTime=-1
  Constant3 : Constant  Value=IIR_DC_F_INIT__PROP  OutDataTypeStr=single  SampleTime=-1
  Constant4 : Constant  Value=IIR_F_SAMPLE__PROP  VectorParams1D=off  OutDataTypeStr=single  SampleTime=-1
  Constant5 : Constant  Value=IIR_IPHASE_F_INIT__PROP  OutDataTypeStr=single  SampleTime=-1
  Constant6 : Constant  Value=FULL_SCALE_VALUE_DC_CURRENT_A__PROP  OutDataTypeStr=single  SampleTime=-1
  Constant7 : Constant  Value=FULL_SCALE_VALUE_PHASE_CURRENT_A__PROP  OutDataTypeStr=single  SampleTime=-1
  Constant8 : Constant  Value=FULL_SCALE_VALUE_DC_VOLTAGE_V__PROP  VectorParams1D=off  OutDataTypeStr=single  SampleTime=-1
  Constant9 : Constant  Value=FULL_SCALE_VALUE_PHASE_VOLTAGE_V__PROP  OutDataTypeStr=single  SampleTime=-1
  Constant94 : Constant  Value=I_TRIP_HW_INIT__PROP  OutDataTypeStr=single  SampleTime=-1
  Data Store Write1 : DataStoreWrite  DataStoreName=oProp  DataStoreElements=oProp.oHw_.fDeadtimeNs_  IndexOptions=Index vector (dialog)  Indices=1  OutputSizes=1
  Data Store Write10 : DataStoreWrite  DataStoreName=oProp  DataStoreElements=oProp.oHw_.uiBLowDelayTicks_  IndexOptions=Index vector (dialog)  Indices=1  OutputSizes=1
  Data Store Write11 : DataStoreWrite  DataStoreName=oProp  DataStoreElements=oProp.oHw_.uiBHighDelayTicks_  IndexOptions=Index vector (dialog)  Indices=1  OutputSizes=1
  Data Store Write12 : DataStoreWrite  DataStoreName=oProp  DataStoreElements=oProp.oHw_.iScalePhaseCurrentLong_  IndexOptions=Index vector (dialog)  Indices=1  OutputSizes=1
  Data Store Write13 : DataStoreWrite  DataStoreName=oProp  DataStoreElements=oProp.oHw_.iScaleDcCurrentLong_  IndexOptions=Index vector (dialog)  Indices=1  OutputSizes=1
  Data Store Write14 : DataStoreWrite  DataStoreName=oProp  DataStoreElements=oProp.oHw_.iScalePhaseVoltageLong_  IndexOptions=Index vector (dialog)  Indices=1  OutputSizes=1
  Data Store Write15 : DataStoreWrite  DataStoreName=oProp  DataStoreElements=oProp.oHw_.iScaleDcVoltageLong_  IndexOptions=Index vector (dialog)  Indices=1  OutputSizes=1
  Data Store Write16 : DataStoreWrite  DataStoreName=oProp  DataStoreElements=oProp.oHw_.iVoltageOffsetPhsLong_  IndexOptions=Index vector (dialog)  Indices=1  OutputSizes=1
  Data Store Write17 : DataStoreWrite  DataStoreName=oProp  DataStoreElements=oProp.oHw_.iVoltageOffsetDcLong_  IndexOptions=Index vector (dialog)  Indices=1  OutputSizes=1
  Data Store Write18 : DataStoreWrite  DataStoreName=oProp  DataStoreElements=oProp.oHw_.fPhaseCurrentSumMaxImbalance_  IndexOptions=Index vector (dialog)  Indices=1  OutputSizes=1
  Data Store Write19 : DataStoreWrite  DataStoreName=oProp  DataStoreElements=oProp.oHw_.iMaxIdenticalSamplesPhaseCurrent_  IndexOptions=Index vector (dialog)  Indices=1  OutputSizes=1
  Data Store Write2 : DataStoreWrite  DataStoreName=oProp  DataStoreElements=oProp.oHw_.fIirUphaseFInit_  IndexOptions=Index vector (dialog)  Indices=1  OutputSizes=1
  Data Store Write3 : DataStoreWrite  DataStoreName=oProp  DataStoreElements=oProp.oHw_.fIirDcFInit_  IndexOptions=Index vector (dialog)  Indices=1  OutputSizes=1
  Data Store Write4 : DataStoreWrite  DataStoreName=oProp  DataStoreElements=oProp.oHw_.fIirFSample_  IndexOptions=Index vector (dialog)  Indices=1  OutputSizes=1
  Data Store Write5 : DataStoreWrite  DataStoreName=oProp  DataStoreElements=oProp.oHw_.fIirIphaseFInit_  IndexOptions=Index vector (dialog)  Indices=1  OutputSizes=1
  Data Store Write6 : DataStoreWrite  DataStoreName=oProp  DataStoreElements=oProp.oHw_.fFullScaleValueDcCurrent_  IndexOptions=Index vector (dialog)  Indices=1  OutputSizes=1
  Data Store Write7 : DataStoreWrite  DataStoreName=oProp  DataStoreElements=oProp.oHw_.fFullScaleValuePhaseCurrent_  IndexOptions=Index vector (dialog)  Indices=1  OutputSizes=1
  Data Store Write8 : DataStoreWrite  DataStoreName=oProp  DataStoreElements=oProp.oHw_.fFullScaleValueDcVoltage_  IndexOptions=Index vector (dialog)  Indices=1  OutputSizes=1
  Data Store Write84 : DataStoreWrite  DataStoreName=oProp  DataStoreElements=oProp.oHw_.fTripLimitHardware_  IndexOptions=Index vector (dialog)  Indices=1  OutputSizes=1
  Data Store Write9 : DataStoreWrite  DataStoreName=oProp  DataStoreElements=oProp.oHw_.fFullScaleValuePhaseVoltage_  IndexOptions=Index vector (dialog)  Indices=1  OutputSizes=1
  wires:
  Constant10/1 -> Data Store Write18/1
  Constant8/1 -> Data Store Write8/1
  Constant1/1 -> Data Store Write1/1
  Constant6/1 -> Data Store Write6/1
  Constant4/1 -> Data Store Write4/1
  Constant9/1 -> Data Store Write9/1
  Constant11/1 -> Data Store Write19/1
  Constant7/1 -> Data Store Write7/1
  Constant94/1 -> Data Store Write84/1
  Constant3/1 -> Data Store Write3/1
  Constant2/1 -> Data Store Write2/1
  Constant5/1 -> Data Store Write5/1
